simulink model "SOGI_FLL"  (R2022b)
settings: Solver=FixedStepAuto  StartTime=0.0  StopTime=1  FixedStep=1e-6  RelTol=1e-3
libraries: spsFourierLib x4, spsVoltageMeasurementLib x1, spspowerguiLib x1, spsControlledVoltageSourceLib x1
settings Model: Creator=XIAO  LastModifiedBy=XIAO
settings DataIOCC: ReturnWorkspaceOutputs=off

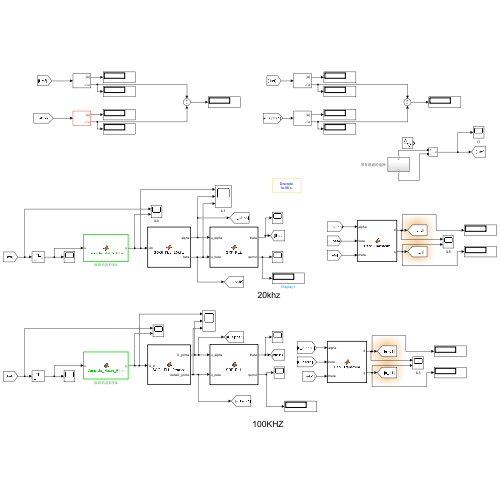
[thumbnail: Simulink's stored preview of the top-level diagram]
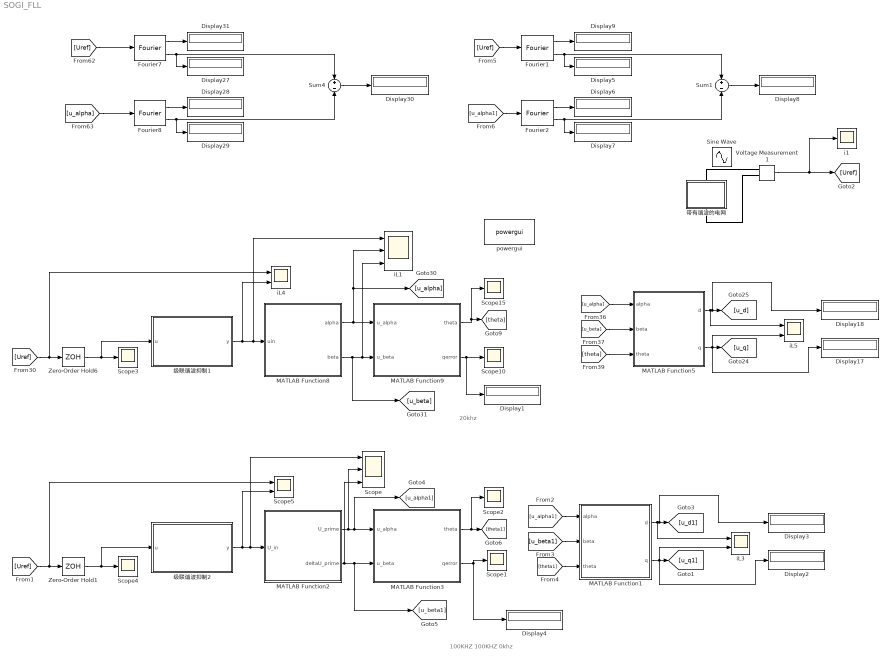
== system SOGI_FLL ==
  note: 20khz
  note: 100KHZ
      |
      | 100KHZ
      | 0khz
  Display{1..9,17..18,27..31} (16 alike) : Display
  Fourier{1..2,7..8} (4 alike) : spsFourierLib/Fourier  Freq=50  n=1  InInit=[0, 0]  Ts=1e-6
  MATLAB Function1 : MATLAB Function  TreatAsAtomicUnit=on
  MATLAB Function2 : MATLAB Function  TreatAsAtomicUnit=on
  MATLAB Function3 : MATLAB Function  TreatAsAtomicUnit=on
  MATLAB Function5 : MATLAB Function  TreatAsAtomicUnit=on
  MATLAB Function8 : MATLAB Function  TreatAsAtomicUnit=on
  MATLAB Function9 : MATLAB Function  TreatAsAtomicUnit=on
  Scope : Scope  NumInputPorts=3
  Scope{1..4,10,15} (6 alike) : Scope
  Scope5 : Scope  NumInputPorts=2
  Sine Wave : Sin  Amplitude=24*sqrt(2)  Frequency=100*pi  SampleTime=0
  Sum1 : Sum  Inputs=+-
  Sum4 : Sum  Inputs=+-
  Voltage Measurement1 : spsVoltageMeasurementLib/Voltage Measurement  PhasorSimulation=off  OutputType=Complex  PSBequivalent=0
  Zero-Order Hold1 : ZeroOrderHold  SampleTime=1e-5
  Zero-Order Hold6 : ZeroOrderHold  SampleTime=5e-5
  i1 : Scope
  iL1 : Scope  NumInputPorts=3
  iL3 : Scope  NumInputPorts=2
  iL4 : Scope  NumInputPorts=2
  iL5 : Scope  NumInputPorts=2
  powergui : spspowerguiLib/powergui  Priority=1  SimulationMode=Discrete  SampleTime=1e-6  frequency=60  Iterations=50  frequencyindice=0  Pbase=100e6  ErrMax=1e-4  UnitsV=kV  UnitsW=MW  buscounter=0  FunctionMessages=off  echomessages=off  EnableUseOfTLC=off  CurrentSourceSwitches=off  DisableSnubberDevices=off  DisableRonSwitches=off  DisableVfSwitches=off  DisplayEquations=off  AutomaticDiscreteSolvers=off  SolverType=Tustin/Backward Euler (TBE)  Interpol=off  ExternalGateDelay=off  methode=off  Ts=100  x0status=blocks  SPID=on  SwTol=0  HookPort=off  NonlinearTolerance=1e-4  nMaxIteration=100  ContinueOnMaxIteration=off  RestoreLinks=warning  ResistiveCurrentMeasurement=off  Frange=[0:2:500]  Ylog=off  Xlog=on  ShowGrid=off  save=off  variable=ZData  structure=0  ZoomFFT=off  StartTime=0.0  cycles=1  DisplayStyle=1  fundamental=60  FreqAxis=off  MaxFrequency=1000  frequencyindicesteady=1  RmsSteady=1  display=off
  带有谐波的电网 : Subsystem
  级联谐波抑制1 : MATLAB Function  TreatAsAtomicUnit=on
  级联谐波抑制2 : MATLAB Function  TreatAsAtomicUnit=on
  wires:
  级联谐波抑制1/1(y) -> iL4/2, iL1/1, MATLAB Function8/1(uin)
  [theta] -> MATLAB Function5/3(theta)
  [u_beta] -> MATLAB Function5/2(beta)
  [Uref] -> iL4/1, Zero-Order Hold6/1
  Zero-Order Hold6/1 -> 级联谐波抑制1/1(u), Scope3/1
  MATLAB Function5/2(q) -> Display17/1, [u_q], iL5/2
  MATLAB Function5/1(d) -> iL5/1, Display18/1, [u_d]
  [u_alpha] -> MATLAB Function5/1(alpha)
  MATLAB Function9/1(theta) -> Scope15/1, [theta]
  MATLAB Function9/2(qerror) -> Scope10/1, Display1/1
  MATLAB Function8/1(alpha) -> [u_alpha], iL1/2, MATLAB Function9/1(u_alpha)
  MATLAB Function8/2(beta) -> MATLAB Function9/2(u_beta), iL1/3, [u_beta]
  Fourier8/1 -> Display28/1
  [u_alpha] -> Fourier8/1
  Fourier8/2 -> Sum4/2, Display29/1
  [Uref] -> Fourier7/1
  Fourier7/2 -> Display27/1, Sum4/1
  Sum4/1 -> Display30/1
  Fourier7/1 -> Display31/1
  MATLAB Function1/1(d) -> iL3/1, Display3/1, [u_d1]
  [u_beta1] -> MATLAB Function1/2(beta)
  [u_alpha1] -> MATLAB Function1/1(alpha)
  MATLAB Function2/1(U_prime) -> Scope/2, MATLAB Function3/1(u_alpha), [u_alpha1]
  MATLAB Function3/1(theta) -> Scope2/1, [theta1]
  级联谐波抑制2/1(y) -> Scope5/2, Scope/1, MATLAB Function2/1(U_in)
  MATLAB Function1/2(q) -> Display2/1, [u_q1], iL3/2
  Zero-Order Hold1/1 -> 级联谐波抑制2/1(u), Scope4/1
  [theta1] -> MATLAB Function1/3(theta)
  MATLAB Function2/2(deltaU_prime) -> Scope/3, [u_beta1], MATLAB Function3/2(u_beta)
  MATLAB Function3/2(qerror) -> Display4/1, Scope1/1
  [Uref] -> Scope5/1, Zero-Order Hold1/1
  Fourier1/1 -> Display9/1
  Sum1/1 -> Display8/1
  [u_alpha1] -> Fourier2/1
  [Uref] -> Fourier1/1
  Fourier2/2 -> Sum1/2, Display7/1
  Fourier2/1 -> Display6/1
  Fourier1/2 -> Display5/1, Sum1/1
  Voltage Measurement1/1 -> i1/1, [Uref]
  connections:
  Voltage Measurement1/LConn1 -- 带有谐波的电网/RConn1
  Voltage Measurement1/LConn2 -- 带有谐波的电网/LConn1

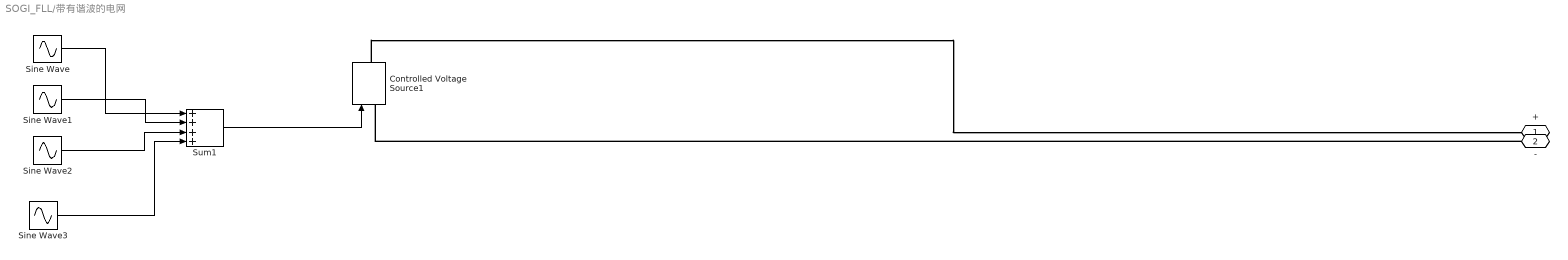
== system SOGI_FLL/带有谐波的电网 ==
  Controlled Voltage Source1 : spsControlledVoltageSourceLib/Controlled Voltage Source  Initialize=off  Source_Type=AC  Amplitude=0  Phase=0  Frequency=0  Measurements=Voltage
  Sine Wave : Sin  Amplitude=24*sqrt(2)  Frequency=100*pi  SampleTime=0
  Sine Wave1 : Sin  Amplitude=0.04*24*sqrt(2)  Frequency=300*pi  SampleTime=0
  Sine Wave2 : Sin  Amplitude=0.03*24*sqrt(2)  Frequency=500*pi  SampleTime=0
  Sine Wave3 : Sin  Amplitude=0.02*24*sqrt(2)  Frequency=700*pi  SampleTime=0
  Sum1 : Sum  Inputs=++++
  + : PMIOPort  Side=Right
  - : PMIOPort  Port=2  Side=Left
  wires:
  Sum1/1 -> Controlled Voltage Source1/1
  Sine Wave1/1 -> Sum1/2
  Sine Wave/1 -> Sum1/1
  Sine Wave3/1 -> Sum1/4
  Sine Wave2/1 -> Sum1/3
  connections:
  -/RConn1 -- Controlled Voltage Source1/LConn1
  Controlled Voltage Source1/RConn1 -- +/RConn1

== matlab function SOGI_FLL/MATLAB Function1 ==
  data: alpha input; d output; beta input; theta input; q output
function [d, q] = Park_Transform(alpha, beta, theta)
% Park变换模块（直接输入SOGI-FLL的theta，无内部积分）
% 输入：
%   alpha - α轴分量（SOGI-FLL的U_prime）
%   beta  - β轴分量（SOGI-FLL的deltaU_prime）
%   theta - 瞬时相位（SOGI-FLL直接输出的theta）
% 输出：
%   d         - d轴（直轴）分量
%   q         - q轴（交轴）分量
%   cos_theta - 相位θ的余弦值（新增输出）
%   sin_theta - 相位θ的正弦值（新增输出）

%% 核心计算
cos_theta = cos(theta);  % 相位θ的余弦值
sin_theta = sin(theta);  % 相位θ的正弦值


% 修正后的 Park 变换公式（d轴对齐同相分量 beta）
d =  alpha * cos_theta + beta * sin_theta;
q = -alpha * sin_theta + beta * cos_theta;
end

== matlab function SOGI_FLL/MATLAB Function2 ==
  settings: updateMethod=DISCRETE
  data: U_in input; U_prime output; deltaU_prime output
function [U_prime, deltaU_prime] = SOGI_FLL_Process(U_in)
% SOGI-FLL for Simulink: 逐点更新，内置相位积分，维护状态记忆
% 输入：U_in   - 当前时刻输入电压（标量）
% 输出：U_prime      - α轴同相输出（标量）
%       deltaU_prime - β轴正交输出（标量）
%       omega0       - 当前角频率（rad/s，标量）
%       theta        - 积分得到的瞬时相位（rad，标量，θ=∫ωdt）

%% 固定参数
dt = 1e-5;               % 仿真步长，必须与Simulink求解器步长一致
K = 1.414;               % SOGI增益
K1 = 0.25;               % 直流消除器增益
gamma = 20;              % FLL增益（你已调至46，加快收敛）
omega0_init = 100*pi;    % 初始角频率（50Hz）
w_max = 2*pi*60;         % 频率上限（60Hz）
w_min = 2*pi*40;         % 频率下限（40Hz）

%% 状态变量持久化（Simulink中必须用persistent）
persistent x1_prev x2_prev x3_prev omega0_prev theta_prev first_run

if isempty(first_run)
    % 首次运行初始化
    x1_prev = 0;
    x2_prev = 0;
    x3_prev = 0;
    omega0_prev = omega0_init;
    theta_prev = 0;       % 相位积分初始值（θ₀=0，匹配输入无初相）
    first_run = false;
end

%% 1. 计算状态导数（逐点，无矩阵）
A11 = -K1 * omega0_prev; A12 = -K1 * omega0_prev; A13 = 0;
A21 = -K  * omega0_prev; A22 = -K  * omega0_prev; A23 = -omega0_prev^2;
A31 = 0;                  A32 = 1;                   A33 = 0;

B1 = K1 * omega0_prev;
B2 = K  * omega0_prev;
B3 = 0;

dx1dt = A11*x1_prev + A12*x2_prev + A13*x3_prev + B1*U_in;
dx2dt = A21*x1_prev + A22*x2_prev + A23*x3_prev + B2*U_in;
dx3dt = A31*x1_prev + A32*x2_prev + A33*x3_prev + B3*U_in;

%% 2. 前向欧拉更新状态
x1_curr = x1_prev + dt * dx1dt;
x2_curr = x2_prev + dt * dx2dt;
x3_curr = x3_prev + dt * dx3dt;

%% 3. FLL频率更新
deltaU = U_in - x1_curr - x2_curr;
deltaU_prime_k = omega0_prev * x3_curr;
epsilon_f = deltaU * deltaU_prime_k;
domega0dt = -gamma * epsilon_f;
omega0_curr = omega0_prev + dt * domega0dt;

% 频率限幅
omega0_curr = max(min(omega0_curr, w_max), w_min);

%% 4. 内置相位积分（梯形积分，精度更高）
% 梯形积分：theta = theta_prev + (当前ω + 前一时刻ω) * dt / 2
theta_curr = theta_prev + (omega0_curr + omega0_prev) * dt / 2;
% 相位归一化（限制在[-π, π]，避免数值溢出）
theta_curr = mod(theta_curr + pi, 2*pi) - pi;

%% 5. 输出
U_prime = x2_curr;
deltaU_prime = omega0_prev * x3_curr;  % 用前一时刻ω₀计算正交分量
omega0 = omega0_curr;
theta = theta_curr;  % 新增相位输出

%% 6. 更新状态，供下一时刻使用
x1_prev = x1_curr;
x2_prev = x2_curr;
x3_prev = x3_curr;
omega0_prev = omega0_curr;
theta_prev = theta_curr;  % 更新相位状态
end

== matlab function SOGI_FLL/MATLAB Function3 ==
  data: u_alpha input; theta output; u_beta input; qerror output
function [theta, qerror] = SRF_PLL(u_alpha, u_beta)
% 同步旋转坐标系锁相环 SRF-PLL（严格匹配框图逻辑）
% 输入
%   u_alpha:  α轴输入信号（对应框图的v'，与电网电压同相）
%   u_beta:   β轴输入信号（对应框图的qv'，与电网电压正交90°）
% 输出
%   theta:    锁相得到的电网相位 [0, 2π)
%   qerror:   q轴相位误差（锁相锁定时趋近于0）
% 适配：仿真步长 Ts=1e-5（10kHz采样），基波频率50Hz

    %% ===================== 1. 固定参数配置 =====================
    Ts = 1e-5;               % 采样时间，必须与全局仿真步长完全一致
    f0 = 50;                  % 电网额定基波频率 (Hz)
    w0 = 2 * pi * f0;        % 额定角频率 (rad/s)
    
    % PI控制器参数（适配10kHz采样，可按需调整）
    kp_pll = 60;              % 比例系数：增大加快锁相响应，过大易振荡
    ki_pll = 5000;            % 积分系数：增大减小稳态相位误差，过大影响稳定性

    %% ===================== 2. 持久变量初始化（仅首次运行执行） =====================
    persistent theta_prev     % 上一拍的锁相相位
    persistent xi_pll         % PI控制器的积分项（抗饱和）
    
    if isempty(theta_prev)
        theta_prev = 0;       % 相位初始值清零
        xi_pll = 0;           % 积分项初始值清零
    end

    %% ===================== 3. αβ/dq 帕克变换（核心鉴相环节） =====================
    % 标准帕克变换矩阵，严格匹配框图逻辑
    % [u_d]   = [ cosθ   sinθ ] [u_alpha]
    % [u_q]     [ -sinθ  cosθ ] [u_beta ]
    cos_theta = cos(theta_prev);
    sin_theta = sin(theta_prev);
    
    u_d = u_alpha * cos_theta + u_beta * sin_theta;  % d轴分量（对应电压幅值）
    u_q = -u_alpha * sin_theta + u_beta * cos_theta; % q轴分量（相位误差）
    
    qerror = u_q; % 输出q轴相位误差，锁相锁定时qerror→0

    %% ===================== 4. PI环路控制器 =====================
    % 位置式PI控制器，带积分抗饱和
    xi_pll = xi_pll + ki_pll * Ts * qerror;  % 积分项更新
    delta_w = kp_pll * qerror + xi_pll;      % 频率偏差量
    w_pll = w0 + delta_w;                     % 锁相得到的实时角频率

    %% ===================== 5. 积分环节（1/s）生成相位 =====================
    % 前向欧拉离散化，对应框图的1/s积分环节
    theta = theta_prev + Ts * w_pll;
    
    % 相位归一化到 [0, 2π)，防止数值溢出
    theta = mod(theta, 2 * pi);

    %% ===================== 6. 更新状态变量（为下一拍迭代准备） =====================
    theta_prev = theta;

end

== matlab function SOGI_FLL/级联谐波抑制2 ==
  data: u input; y output
function y = Cascade_Notch_Filter(u)
% 级联陷波滤波器：滤除3/5/7次固定频率谐波（150/250/350Hz）
% 输入u：待滤波的标量信号
% 输出y：滤波后的标量信号
% 适配：20kHz采样率（Ts=5e-5），和你的控制环完全对齐

    persistent x3_1 x3_2 x5_1 x5_2 x7_1 x7_2 first_run
    persistent b3_0 b3_1 b3_2 a3_1 a3_2
    persistent b5_0 b5_1 b5_2 a5_1 a5_2
    persistent b7_0 b7_1 b7_2 a7_1 a7_2

    %% ===================== 1. 初始化：仅首次运行 =====================
    if isempty(first_run)
        % --- 固定参数 ---
        Fs = 1e5;          % 采样频率 100kHz
        Ts = 1/Fs;            % 采样周期 1e-5s
        wc = 10;              % 截止角频率 25 rad/s
        
        % 目标谐波频率
        w3 = 2*pi*150;  % 3次谐波 150Hz
        w5 = 2*pi*250;  % 5次谐波 250Hz
        w7 = 2*pi*350;  % 7次谐波 350Hz

        % --- Tustin变换预计算系数 ---
        k = 2/Ts;
        k2 = k*k;

        % --- 3次滤波器系数 ---
        [b3_0, b3_1, b3_2, a3_1, a3_2] = calc_coeff(w3, wc, k, k2);
        % --- 5次滤波器系数 ---
        [b5_0, b5_1, b5_2, a5_1, a5_2] = calc_coeff(w5, wc, k, k2);
        % --- 7次滤波器系数 ---
        [b7_0, b7_1, b7_2, a7_1, a7_2] = calc_coeff(w7, wc, k, k2);

        % --- 显式初始化状态变量为标量 ---
        x3_1 = 0; x3_2 = 0;
        x5_1 = 0; x5_2 = 0;
        x7_1 = 0; x7_2 = 0;
        
        first_run = 1;
    end

    %% ===================== 2. 级联滤波计算（显式差分方程） =====================
    % --- 第1级：3次谐波滤波 ---
    y3 = b3_0*u + x3_1;
    x3_1_next = b3_1*u - a3_1*y3 + x3_2;
    x3_2_next = b3_2*u - a3_2*y3;
    
    % --- 第2级：5次谐波滤波 ---
    y5 = b5_0*y3 + x5_1;
    x5_1_next = b5_1*y3 - a5_1*y5 + x5_2;
    x5_2_next = b5_2*y3 - a5_2*y5;
    
    % --- 第3级：7次谐波滤波 ---
    y7 = b7_0*y5 + x7_1;
    x7_1_next = b7_1*y5 - a7_1*y7 + x7_2;
    x7_2_next = b7_2*y5 - a7_2*y7;
    
    % --- 更新状态变量 ---
    x3_1 = x3_1_next; x3_2 = x3_2_next;
    x5_1 = x5_1_next; x5_2 = x5_2_next;
    x7_1 = x7_1_next; x7_2 = x7_2_next;
    
    % --- 最终输出 ---
    y = y7;

end

%% ===================== 局部函数：预计算滤波器系数 =====================
function [b0, b1, b2, a1, a2] = calc_coeff(wn, wc, k, k2)
    % 连续域：G(s) = (s^2 + wn^2) / (s^2 + 2*wc*s + wn^2)
    % Tustin离散化：s = k*(z-1)/(z+1)
    
    % 连续域系数
    num_b0 = 1; num_b1 = 0; num_b2 = wn^2;
    den_a0 = 1; den_a1 = 2*wc; den_a2 = wn^2;
    
    % 离散化计算
    B0 = num_b0*k2 + num_b1*k + num_b2;
    B1 = 2*num_b2 - 2*num_b0*k2;
    B2 = num_b0*k2 - num_b1*k + num_b2;
    
    A0 = den_a0*k2 + den_a1*k + den_a2;
    A1 = 2*den_a2 - 2*den_a0*k2;
    A2 = den_a0*k2 - den_a1*k + den_a2;
    
    % 归一化（a0=1）
    b0 = B0 / A0;
    b1 = B1 / A0;
    b2 = B2 / A0;
    a1 = A1 / A0;
    a2 = A2 / A0;
end

== matlab function SOGI_FLL/MATLAB Function5 ==
  data: alpha input; d output; beta input; theta input; q output
function [d, q] = Park_Transform(alpha, beta, theta)
% Park变换模块（直接输入SOGI-FLL的theta，无内部积分）
% 输入：
%   alpha - α轴分量（SOGI-FLL的U_prime）
%   beta  - β轴分量（SOGI-FLL的deltaU_prime）
%   theta - 瞬时相位（SOGI-FLL直接输出的theta）
% 输出：
%   d         - d轴（直轴）分量
%   q         - q轴（交轴）分量
%   cos_theta - 相位θ的余弦值（新增输出）
%   sin_theta - 相位θ的正弦值（新增输出）

%% 核心计算
cos_theta = cos(theta);  % 相位θ的余弦值
sin_theta = sin(theta);  % 相位θ的正弦值


% 修正后的 Park 变换公式（d轴对齐同相分量 beta）
d =  alpha * cos_theta + beta * sin_theta;
q = -alpha * sin_theta + beta * cos_theta;
end

== matlab function SOGI_FLL/MATLAB Function8 ==
  settings: updateMethod=DISCRETE
  data: uin input; alpha output; beta output
function [alpha, beta] = SOGI_FLL_20kHz(uin)
% 严格对应你的 m 文件：20kHz 双线性 PI-FLL
% 输入：uin   单相电压
% 输出：alpha 同相输出 uα = x2
%      beta  正交输出 uβ = omega0*x3

%% 固定参数（和你的m文件完全一致）
dt = 5e-5;
K  = 1.414;
K1 = 0.25;
gamma_p =30;
gamma_i =500;
w_max = 2*pi*60;
w_min = 2*pi*40;

%% 状态持久化
persistent x1_prev x2_prev x3_prev omega0_prev U_prev integral_f first_run;
if isempty(first_run)
    x1_prev = 0;
    x2_prev = 0;
    x3_prev = 0;
    omega0_prev = 2*pi*50;
    U_prev = uin;
    integral_f = 0;
    first_run = false;
end

%% 1. 当前输入
U_curr = uin;
omega0_prev_local = omega0_prev;

%% 2. 频率预畸变
omega_pre = (2/dt) * tan(omega0_prev_local * dt / 2);

%% 3. 状态矩阵 A, B
A_mat = [
    -K1*omega_pre, -K1*omega_pre, 0;
    -K*omega_pre,  -K*omega_pre,  -omega_pre^2;
    0,              1,              0
];
B_mat = [
    K1*omega_pre;
    K*omega_pre;
    0
];

%% 4. 双线性变换
I_mat = eye(3);
M1 = I_mat - (dt/2)*A_mat;
M2 = I_mat + (dt/2)*A_mat;
U_avg = U_curr + U_prev;

x_prev_vec = [x1_prev; x2_prev; x3_prev];
x_curr_vec = M1 \ (M2 * x_prev_vec + (dt/2)*B_mat * U_avg);

x1_curr = x_curr_vec(1);
x2_curr = x_curr_vec(2);
x3_curr = x_curr_vec(3);

%% 5. PI-FLL 频率环
deltaU = U_curr - x1_curr - x2_curr;
deltaU_prime_val = omega0_prev_local * x3_curr;
epsilon_f = deltaU * deltaU_prime_val;

integral_f = integral_f + epsilon_f * dt;
domega0dt = -gamma_p * epsilon_f - gamma_i * integral_f;
omega0_curr = omega0_prev_local + dt * domega0dt;

% 频率限幅
omega0_curr = max(min(omega0_curr, w_max), w_min);

%% 6. 输出 alpha beta
alpha = x2_curr;
beta  = omega0_curr * x3_curr;

%% 7. 更新状态
x1_prev = x1_curr;
x2_prev = x2_curr;
x3_prev = x3_curr;
omega0_prev = omega0_curr;
U_prev = U_curr;

end

== matlab function SOGI_FLL/MATLAB Function9 ==
  data: u_alpha input; theta output; u_beta input; qerror output
function [theta, qerror] = SRF_PLL(u_alpha, u_beta)
% 同步旋转坐标系锁相环 SRF-PLL
% 【已修改为：纯自适应频率版本 → 和你主循环PLL完全一致】
% 输入：u_alpha, u_beta
% 输出：theta 锁相相位, qerror q分量（趋近0）

    %% ===================== 1. 固定参数 =====================
    Ts = 5e-5;               % 20kHz 采样步长（必须匹配）
    
    % PI参数（和你主循环一致）
    kp_pll = 200;
    ki_pll = 7000;

    %% ===================== 2. 持久变量 =====================
    persistent theta_prev
    persistent integral_pll
    
    if isempty(theta_prev)
        theta_prev = 0;
        integral_pll = 0;
    end

    %% ===================== 3. Park 变换 =====================
    cos_theta = cos(theta_prev);
    sin_theta = sin(theta_prev);
    
    u_d =  u_alpha * cos_theta + u_beta * sin_theta;
    u_q = -u_alpha * sin_theta + u_beta * cos_theta;
    
    qerror = u_q;  % q分量（锁相成功→0）

    %% ===================== 4. PI控制器（我的版本：直接输出ω） =====================
    integral_pll = integral_pll + qerror * Ts;          % 积分
    omega_pll    = kp_pll * qerror + ki_pll * integral_pll; % 直接输出角频率

    %% ===================== 5. 积分生成相位 =====================
    theta = theta_prev + omega_pll * Ts;

    %% ===================== 6. 相位归一化（±π） =====================
    if theta > pi
        theta = theta - 2*pi;
    elseif theta < -pi
        theta = theta + 2*pi;
    end

    %% ===================== 7. 更新状态 =====================
    theta_prev = theta;
end

== matlab function SOGI_FLL/级联谐波抑制1 ==
  data: u input; y output
function y = Cascade_Notch_Filter(u)
% 级联陷波滤波器：滤除3/5/7次固定频率谐波（150/250/350Hz）
% 输入u：待滤波的标量信号
% 输出y：滤波后的标量信号
% 适配：20kHz采样率（Ts=5e-5），和你的控制环完全对齐

    persistent x3_1 x3_2 x5_1 x5_2 x7_1 x7_2 first_run
    persistent b3_0 b3_1 b3_2 a3_1 a3_2
    persistent b5_0 b5_1 b5_2 a5_1 a5_2
    persistent b7_0 b7_1 b7_2 a7_1 a7_2

    %% ===================== 1. 初始化：仅首次运行 =====================
    if isempty(first_run)
        % --- 固定参数 ---
        Fs = 2e4;          % 采样频率 20kHz
        Ts = 1/Fs;            % 采样周期 5e-5s
        wc = 10;              % 截止角频率 25 rad/s
        
        % 目标谐波频率
        w3 = 2*pi*150;  % 3次谐波 150Hz
        w5 = 2*pi*250;  % 5次谐波 250Hz
        w7 = 2*pi*350;  % 7次谐波 350Hz

        % --- Tustin变换预计算系数 ---
        k = 2/Ts;
        k2 = k*k;

        % --- 3次滤波器系数 ---
        [b3_0, b3_1, b3_2, a3_1, a3_2] = calc_coeff(w3, wc, k, k2);
        % --- 5次滤波器系数 ---
        [b5_0, b5_1, b5_2, a5_1, a5_2] = calc_coeff(w5, wc, k, k2);
        % --- 7次滤波器系数 ---
        [b7_0, b7_1, b7_2, a7_1, a7_2] = calc_coeff(w7, wc, k, k2);

        % --- 显式初始化状态变量为标量 ---
        x3_1 = 0; x3_2 = 0;
        x5_1 = 0; x5_2 = 0;
        x7_1 = 0; x7_2 = 0;
        
        first_run = 1;
    end

    %% ===================== 2. 级联滤波计算（显式差分方程） =====================
    % --- 第1级：3次谐波滤波 ---
    y3 = b3_0*u + x3_1;
    x3_1_next = b3_1*u - a3_1*y3 + x3_2;
    x3_2_next = b3_2*u - a3_2*y3;
    
    % --- 第2级：5次谐波滤波 ---
    y5 = b5_0*y3 + x5_1;
    x5_1_next = b5_1*y3 - a5_1*y5 + x5_2;
    x5_2_next = b5_2*y3 - a5_2*y5;
    
    % --- 第3级：7次谐波滤波 ---
    y7 = b7_0*y5 + x7_1;
    x7_1_next = b7_1*y5 - a7_1*y7 + x7_2;
    x7_2_next = b7_2*y5 - a7_2*y7;
    
    % --- 更新状态变量 ---
    x3_1 = x3_1_next; x3_2 = x3_2_next;
    x5_1 = x5_1_next; x5_2 = x5_2_next;
    x7_1 = x7_1_next; x7_2 = x7_2_next;
    
    % --- 最终输出 ---
    y = y7;

end

%% ===================== 局部函数：预计算滤波器系数 =====================
function [b0, b1, b2, a1, a2] = calc_coeff(wn, wc, k, k2)
    % 连续域：G(s) = (s^2 + wn^2) / (s^2 + 2*wc*s + wn^2)
    % Tustin离散化：s = k*(z-1)/(z+1)
    
    % 连续域系数
    num_b0 = 1; num_b1 = 0; num_b2 = wn^2;
    den_a0 = 1; den_a1 = 2*wc; den_a2 = wn^2;
    
    % 离散化计算
    B0 = num_b0*k2 + num_b1*k + num_b2;
    B1 = 2*num_b2 - 2*num_b0*k2;
    B2 = num_b0*k2 - num_b1*k + num_b2;
    
    A0 = den_a0*k2 + den_a1*k + den_a2;
    A1 = 2*den_a2 - 2*den_a0*k2;
    A2 = den_a0*k2 - den_a1*k + den_a2;
    
    % 归一化（a0=1）
    b0 = B0 / A0;
    b1 = B1 / A0;
    b2 = B2 / A0;
    a1 = A1 / A0;
    a2 = A2 / A0;
end
